simulink model "microgrid"  (R2023b)
settings: Solver=VariableStepAuto  StartTime=0.0  StopTime=24*60*60  RelTol=1e-3
PreLoadFcn:
  | microgrid_parameters
values from neighbouring files (symbols this model uses):
  PV = photovoltaic_parameters    [microgrid_parameters.m]
undefined symbols (not defined in the file or in its folder): BUS, URFC
libraries: fl_lib x19, ee_lib x5, nesl_utility x4, SignalEditorBlockLib x1
settings Model: Creator=michaelfsb  LastModifiedBy=michaelfsb
settings DebuggingCC: IgnoredZcDiagnostic=error

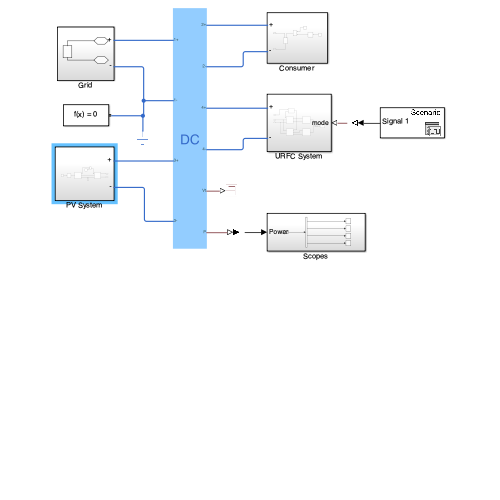
[thumbnail: Simulink's stored preview of the top-level diagram]
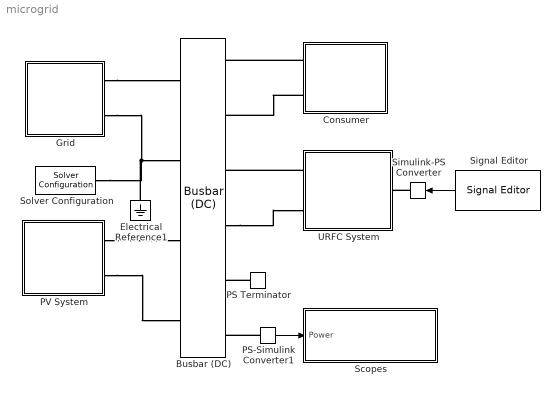
== system microgrid ==
  Busbar (DC) : ee_lib/Connectors & References/Busbar (DC)  n_nodes=ee.enum.connectors.busbar_number_of_connections.four  VRated=BUS.Voltage V  measurement_type=ee.enum.measurementType.instantaneous  averaging_period=1e-2 s  show_ps=ee.enum.connectors.busbar_measurement.true
      settings: InternalSimscapePortConfiguration="{\"Bottom\":[],\"Left\":[{\"id\":\"p1\",\"label\":\"1+\",\"type\":\"foundation.electrical.electrical\"},{\"id\":\"n1\",\"label\":\"1-\",\"type\":\"foundation.electrical.electrical\"},{\"id\":\"p3\",\"label\":\"3+\",\"type\":\"foundation.electrical.electrical\"},{\"id\":\"n3\",\"label\":\"3-\",\"type\":\"foundation.electrical.electrical\"}],\"Right\":[{\"id\":\"p2\",\"label\":\"2+\",\"type\":\"foundation.electrical.electrical\"},{\"id\":\"n2\",\"label\":\"2-\",\"type\":\"foundation.electrical.electrical\"},{\"id\":\"p4\",\"label\":\"4+\",\"type\":\"foundation.electrical.electrical\"},{\"id\":\"n4\",\"label\":\"4-\",\"type\":\"foundation.electrical.electrical\"},{\"id\":\"Vt_ps\",\"label\":\"Vt\",\"type\":\"output\"},{\"id\":\"P4_ps\",\"label\":\"P\",\"type\":\"output\"}],\"Top\":[]}"
  Consumer : Subsystem
  Electrical Reference1 : fl_lib/Electrical/Electrical Elements/Electrical Reference
  Grid : Subsystem
      settings: PortSchema="{\"entries\":[{\"content\":{\"sides\":[{\"content\":{},\"type\":\"ConnectorPlacement.EquallySpacedRectSide\",\"uuid\":\"7d3e1531-3ac3-48d1-8d53-8dc071a39518\"},{\"content\":{\"side\":\"RIGHT\"},\"type\":\"ConnectorPlacement.EquallySpacedRectSide\",\"uuid\":\"25b50bd9-2b9f-4527-8fc7-8205feed0a4d\"},{\"content\":{\"connectorIds\":[\"LConn1\",\"LConn2\"],\"side\":\"TOP\"},\"type\":\"ConnectorPlacement.EquallySpacedRectSide\",\"uuid\":\"ec9d499b-92d3-45f6-91a8-3c7a2a7323b8\"}]},\"type\":\"ConnectorPlacement.EquallySpacedConnector\",\"uuid\":\"21f9d016-eefb-40e7-aeda-3b0d2900fe93\"}],\"packageUris\":[\"http://schema.mathworks.com/mf0/Connector/R2020b\"],\"version\":\"1.0\"}"
  PS Terminator : fl_lib/Physical Signals/Sinks/PS Terminator
  PS-Simulink Converter1 : nesl_utility/PS-Simulink Converter  PhysicalDomain=network_engine_domain  SubClassName=ps_output  LeftPortType=input  RightPortType=output  PseudoPeriodic=off  Frequencies=[]  VectorFormat=inherit  Unit=inherit  AffineConversion=off
  PV System : Subsystem
      settings: PortSchema="{\"entries\":[{\"content\":{\"sides\":[{\"content\":{},\"type\":\"ConnectorPlacement.EquallySpacedRectSide\",\"uuid\":\"7d3e1531-3ac3-48d1-8d53-8dc071a39518\"},{\"content\":{\"side\":\"RIGHT\"},\"type\":\"ConnectorPlacement.EquallySpacedRectSide\",\"uuid\":\"25b50bd9-2b9f-4527-8fc7-8205feed0a4d\"},{\"content\":{\"connectorIds\":[\"LConn1\",\"LConn2\"],\"side\":\"TOP\"},\"type\":\"ConnectorPlacement.EquallySpacedRectSide\",\"uuid\":\"ec9d499b-92d3-45f6-91a8-3c7a2a7323b8\"}]},\"type\":\"ConnectorPlacement.EquallySpacedConnector\",\"uuid\":\"21f9d016-eefb-40e7-aeda-3b0d2900fe93\"}],\"packageUris\":[\"http://schema.mathworks.com/mf0/Connector/R2020b\"],\"version\":\"1.0\"}"
  Scopes : Subsystem
  Signal Editor : SignalEditorBlockLib/Signal Editor  FileName=op_mode_siginal.mat  ActiveScenario=Scenario  ActiveSignal=Signal 1  IsBus=off  OutputBusObjectStr=Bus: BusObject  SampleTime=0  Interpolate=off  ZeroCross=off  OutputAfterFinalValue=Setting to zero  Unit=inherit  PreserveSignalName=on  ApplySigPropsToAllScenarios=on  ApplySigPropsToAllSignals=off
  Simulink-PS Converter : nesl_utility/Simulink-PS Converter  PhysicalDomain=network_engine_domain  SubClassName=ps_input  LeftPortType=input  RightPortType=output  PseudoPeriodic=off  Frequencies=[]  NoiseDistribution=none  NoiseParameters=[]  Unit=1  AffineConversion=off  FilteringAndDerivatives=provide  SimscapeFilterOrder=1  InputFilterTimeConstant=0.001  UdotUserProvided=0
  Solver Configuration : nesl_utility/Solver Configuration  PhysicalDomain=network_engine_domain  SubClassName=solver  LeftPortType=input  RightPortType=generic  Tones=[]  Harmonics=[]  SimulateNoise=off  Profile=off  UseLocalSampling=off  EnableSwitchedLinearOptims=on  FrequencyDomain=off  UseCCode=off  RelTol=0.001  AbsTol=0.001  MinStep=1e-09  ToWorkspace=off  RevertToSquareIcSolve=off  NumHomotopyIterations=100  PhasorMode=off  PhasorModeNumHarmonics=1  ConsistencySolver=NEWTON_XTOL_AFTER_FTOL  IndexReductionMethod=DerivativeReplacement  DoDC=off  ResidualTolerance=1e-09  ConsistencyTolSource=GLOBAL  ConsistencyAbsTol=0.001  ConsistencyRelTol=0.001  ConsistencyTolFactor=0.001  UseLocalSolver=off  LocalSolverChoice=NE_BACKWARD_EULER_ADVANCER  ResolveIndetEquations=on  FunctionEvalNumThread=1  LocalSolverSampleTime=0.001  DoFixedCost=off  MaxNonlinIter=3  MaxModeIter=2  ComputeImpulses=off  ImpulseIterations=2  LinearAlgebra=auto  LinearAlgebraNumThread=0  EquationFormulation=NE_TIME_EF  DelaysMemoryBudget=1024  AutomaticFiltering=on  FilteringTimeConstant=0.001  PartitionStorageMethod=AS_NEEDED  PartitionMemoryBudget=1024  PartitionMethod=ROBUST  MultibodyUseLocalSolver=off  MultibodyLocalSolverChoice=ODE1  MultibodyLocalSolverSampleTime=0.001
  URFC System : Subsystem
  wires:
  PS-Simulink Converter1/1 -> Scopes/1(Power)
  Signal Editor/1 -> Simulink-PS Converter/1
  connections:
  Grid/LConn1 -- Busbar (DC)/LConn1
  PV System/LConn1 -- Busbar (DC)/LConn3
  Consumer/LConn1 -- Busbar (DC)/RConn1
  PV System/LConn2 -- Busbar (DC)/LConn4
  Grid/LConn2 -- Solver Configuration/RConn1 -- Electrical Reference1/LConn1 -- Busbar (DC)/LConn2
  Consumer/LConn2 -- Busbar (DC)/RConn2
  PS-Simulink Converter1/LConn1 -- Busbar (DC)/RConn6
  PS Terminator/LConn1 -- Busbar (DC)/RConn5
  URFC System/RConn1 -- Busbar (DC)/RConn3
  Simulink-PS Converter/RConn1 -- URFC System/LConn1
  Busbar (DC)/RConn4 -- URFC System/RConn2

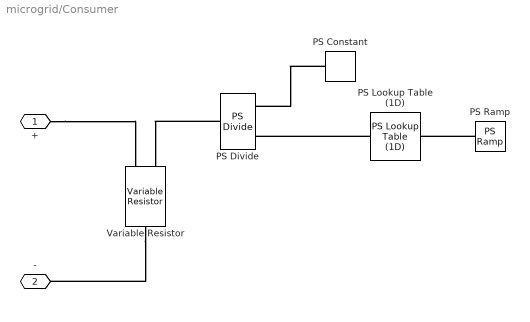
== system microgrid/Consumer ==
  PS Constant : fl_lib/Physical Signals/Sources/PS Constant  constant=BUS.Voltage^2 V^2
  PS Divide : fl_lib/Physical Signals/Functions/PS Divide
  PS Lookup Table (1D) : fl_lib/Physical Signals/Lookup Tables/PS Lookup Table (1D)  x=power_demand.time  f=power_demand.data W  interp_method=simscape.enum.interpolation.linear  extrap_method=simscape.enum.extrapolation.linear
  PS Ramp : fl_lib/Physical Signals/Sources/PS Ramp  slope=1 1/s  start_time=0 s  initial_output=0
  Variable Resistor : fl_lib/Electrical/Electrical Elements/Variable Resistor  Rmin=0 Ohm  thermalEnable=false  thermal_mass=1 J/K  i_specify=off  i_priority=None  i=0 A  i_nominal_specify=off  i_nominal_unit=A  i_nominal_value=1  v_specify=off  v_priority=None  v=0 V  v_nominal_specify=off  v_nominal_unit=V  v_nominal_value=1  T_specify=off  T_priority=None  T=300 K  T_nominal_specify=off  T_nominal_unit=K  T_nominal_value=1
  + : PMIOPort  Side=Left
  - : PMIOPort  Port=2  Side=Left
  connections:
  Variable Resistor/RConn1 -- -/RConn1
  PS Ramp/RConn1 -- PS Lookup Table (1D)/LConn1
  PS Constant/RConn1 -- PS Divide/LConn1
  PS Divide/RConn1 -- Variable Resistor/LConn1
  +/RConn1 -- Variable Resistor/LConn2
  PS Lookup Table (1D)/RConn1 -- PS Divide/LConn2

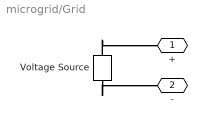
== system microgrid/Grid ==
  Voltage Source : ee_lib/Sources/Voltage Source  dc_voltage=BUS.Voltage V  ac_voltage=0 V  ac_shift=0 rad  ac_frequency=60 Hz  noise_mode=ee.enum.sources.noise.Disabled  PSD=0 V^2/Hz  sample_time=1e-3 s  repeatability=ee.enum.sources.repeatability.NotRepeatable  user_seed=0  auto_seed=414269032  i_specify=off  i_priority=None  i=0 A  i_nominal_specify=off  i_nominal_unit=A  i_nominal_value=1  v_specify=off  v_priority=None  v=0 V  v_nominal_specify=off  v_nominal_unit=V  v_nominal_value=1
  + : PMIOPort  Side=Left
  - : PMIOPort  Port=2  Side=Left
  connections:
  Voltage Source/LConn1 -- +/RConn1
  Voltage Source/RConn1 -- -/RConn1

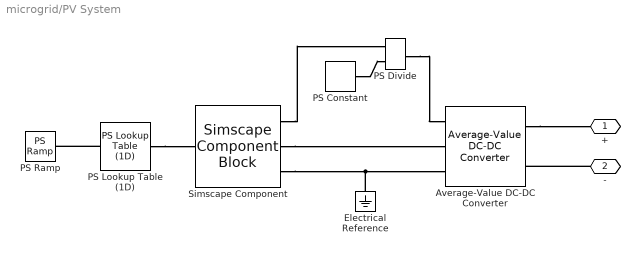
== system microgrid/PV System ==
  Average-Value DC-DC Converter : ee_lib/Semiconductors & Converters/Converters/Average-Value DC-DC Converter  control_option=ee.enum.converters.controlinput.current  converter_type=ee.enum.converters.dcdctype.boost  efficiency_option=ee.enum.converters.efficiency.constant  efficiency_fixed=100  i_vec=[0, 2, 5] A  efficiency_vec=[90, 95, 98]
      settings: InternalSimscapePortConfiguration="{\"Bottom\":[],\"Left\":[{\"id\":\"Iref\",\"label\":\"Iref\",\"type\":\"input\"},{\"id\":\"p1\",\"label\":\"1+\",\"type\":\"foundation.electrical.electrical\"},{\"id\":\"n1\",\"label\":\"1-\",\"type\":\"foundation.electrical.electrical\"}],\"Right\":[{\"id\":\"p2\",\"label\":\"2+\",\"type\":\"foundation.electrical.electrical\"},{\"id\":\"n2\",\"label\":\"2-\",\"type\":\"foundation.electrical.electrical\"}],\"Top\":[]}"
  Electrical Reference : fl_lib/Electrical/Electrical Elements/Electrical Reference
  PS Constant : fl_lib/Physical Signals/Sources/PS Constant  constant=BUS.Voltage V
  PS Divide : fl_lib/Physical Signals/Functions/PS Divide
  PS Lookup Table (1D) : fl_lib/Physical Signals/Lookup Tables/PS Lookup Table (1D)  x=radiation.time  f=radiation.data  interp_method=simscape.enum.interpolation.linear  extrap_method=simscape.enum.extrapolation.linear
  PS Ramp : fl_lib/Physical Signals/Sources/PS Ramp  slope=1 1/s  start_time=0 s  initial_output=0
  Simscape Component : SimscapeComponentBlock  SourceFile=pv_panel  ComponentPath=pv_panel  ComponentVariants="[\"pv_panel\"]"  ComponentVariantNames="[\"pv_panel\"]"  ClassName=pv_panel  SchemaVersion=1  Nps=PV.N_ps  Nss=PV.N_ss  T=PV.T_ps K  Tr=PV.Tr K  Isc=PV.Isc A  Kl=PV.Kl A/K  Ior=PV.Ior A  Ego=PV.Ego V  A=PV.A  v_specify=off  v_priority=None  v=0 V  v_nominal_specify=off  v_nominal_unit=V  v_nominal_value=1  i_specify=off  i_priority=None  i=0 A  i_nominal_specify=off  i_nominal_unit=A  i_nominal_value=1
      settings: CopyFcn=simscape.engine.sli.internal.componentblockcallback(gcbh,'COPY')  PreCopyFcn=simscape.engine.sli.internal.componentblockcallback(gcbh,'PRECOPY')  PreDeleteFcn=simscape.engine.sli.internal.componentblockcallback(gcbh,'PREDELETE')  InternalSimscapePortConfiguration="{\"Bottom\":[],\"Left\":[{\"id\":\"lambda\",\"label\":\"l\",\"type\":\"input\"}],\"Right\":[{\"id\":\"p_mppt\",\"label\":\"p\",\"type\":\"output\"},{\"id\":\"p\",\"label\":\"+\",\"type\":\"foundation.electrical.electrical\"},{\"id\":\"n\",\"label\":\"-\",\"type\":\"foundation.electrical.electrical\"}],\"Top\":[]}"
      mask Type: pv_panel
  + : PMIOPort  Side=Left
  - : PMIOPort  Port=2  Side=Left
  connections:
  Electrical Reference/LConn1 -- Average-Value DC-DC Converter/LConn3 -- Simscape Component/RConn3
  PS Lookup Table (1D)/LConn1 -- PS Ramp/RConn1
  PS Lookup Table (1D)/RConn1 -- Simscape Component/LConn1
  -/RConn1 -- Average-Value DC-DC Converter/RConn2
  Average-Value DC-DC Converter/RConn1 -- +/RConn1
  Simscape Component/RConn2 -- Average-Value DC-DC Converter/LConn2
  Simscape Component/RConn1 -- PS Divide/LConn1
  PS Constant/RConn1 -- PS Divide/LConn2
  PS Divide/RConn1 -- Average-Value DC-DC Converter/LConn1

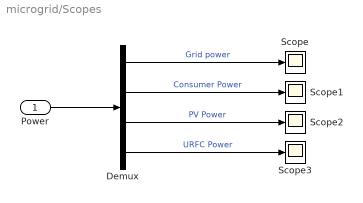
== system microgrid/Scopes ==
  Power : Inport
  Demux : Demux
  Scope{,1..3} (4 alike) : Scope
  wires:
  Power/1 -> Demux/1
  Demux/1 -> Scope/1  "Grid power"
  Demux/4 -> Scope3/1  "URFC Power"
  Demux/2 -> Scope1/1  "Consumer Power"
  Demux/3 -> Scope2/1  "PV Power"

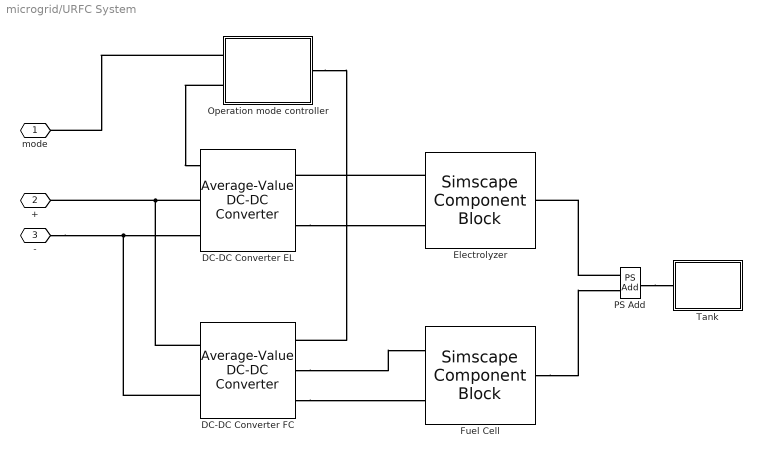
== system microgrid/URFC System ==
  DC-DC Converter EL : ee_lib/Semiconductors & Converters/Converters/Average-Value DC-DC Converter  control_option=ee.enum.converters.controlinput.current  converter_type=ee.enum.converters.dcdctype.buck  efficiency_option=ee.enum.converters.efficiency.constant  efficiency_fixed=100  i_vec=[0, 2, 5] A  efficiency_vec=[90, 95, 98]
      settings: LogSimulationData=on  InternalSimscapePortConfiguration="{\"Bottom\":[],\"Left\":[{\"id\":\"Iref\",\"label\":\"Iref\",\"type\":\"input\"},{\"id\":\"p1\",\"label\":\"1+\",\"type\":\"foundation.electrical.electrical\"},{\"id\":\"n1\",\"label\":\"1-\",\"type\":\"foundation.electrical.electrical\"}],\"Right\":[{\"id\":\"p2\",\"label\":\"2+\",\"type\":\"foundation.electrical.electrical\"},{\"id\":\"n2\",\"label\":\"2-\",\"type\":\"foundation.electrical.electrical\"}],\"Top\":[]}"
  DC-DC Converter FC : ee_lib/Semiconductors & Converters/Converters/Average-Value DC-DC Converter  control_option=ee.enum.converters.controlinput.current  converter_type=ee.enum.converters.dcdctype.buck  efficiency_option=ee.enum.converters.efficiency.constant  efficiency_fixed=100  i_vec=[0, 2, 5] A  efficiency_vec=[90, 95, 98]
      settings: LogSimulationData=on  InternalSimscapePortConfiguration="{\"Bottom\":[],\"Left\":[{\"id\":\"Iref\",\"label\":\"Iref\",\"type\":\"input\"},{\"id\":\"p1\",\"label\":\"1+\",\"type\":\"foundation.electrical.electrical\"},{\"id\":\"n1\",\"label\":\"1-\",\"type\":\"foundation.electrical.electrical\"}],\"Right\":[{\"id\":\"p2\",\"label\":\"2+\",\"type\":\"foundation.electrical.electrical\"},{\"id\":\"n2\",\"label\":\"2-\",\"type\":\"foundation.electrical.electrical\"}],\"Top\":[]}"
  Electrolyzer : SimscapeComponentBlock  SourceFile=urfc_electrolyzer  ComponentPath=urfc_electrolyzer  ComponentVariants="[\"urfc_electrolyzer\"]"  ComponentVariantNames="[\"urfc_electrolyzer\"]"  ClassName=urfc_electrolyzer  SchemaVersion=1  N_cells=10  A_cell=100 cm^2  alpha=0.5  E_rev_0=1.23 V  I_loss_internal=0.008 A/cm^2  I_o_anode=0.15 A/cm^2  I_o_cathode=1.5e-4 A/cm^2  R_ion=0.01 Ohm*cm^2  R_CR=0.03 Ohm*cm^2  R_elect=0 Ohm*cm^2  I_limit_anode=15 A/cm^2  I_limit_cathode=2.5 A/cm^2  A_anodo=0.0304 V  A_catodo=0.0507 V  T=353.15 K  R_gas=8.3145 J/(K*mol)  F_constant=96485 C/mol  n_electrons=2  i_specify=off  i_priority=None  i=0 A  i_nominal_specify=off  i_nominal_unit=A  i_nominal_value=1  v_specify=off  v_priority=None  v=0 V  v_nominal_specify=off  v_nominal_unit=V  v_nominal_value=1
      settings: CopyFcn=simscape.engine.sli.internal.componentblockcallback(gcbh,'COPY')  PreCopyFcn=simscape.engine.sli.internal.componentblockcallback(gcbh,'PRECOPY')  PreDeleteFcn=simscape.engine.sli.internal.componentblockcallback(gcbh,'PREDELETE')  InternalSimscapePortConfiguration="{\"Bottom\":[],\"Left\":[{\"id\":\"p\",\"label\":\"+\",\"type\":\"foundation.electrical.electrical\"},{\"id\":\"n\",\"label\":\"-\",\"type\":\"foundation.electrical.electrical\"}],\"Right\":[{\"id\":\"h2\",\"label\":\"H2\",\"type\":\"output\"}],\"Top\":[]}"
      mask Type: Electrolyzer mode model of a URFC
  Fuel Cell : SimscapeComponentBlock  SourceFile=urfc_fuel_cell  ComponentPath=urfc_fuel_cell  ComponentVariants="[\"urfc_fuel_cell\"]"  ComponentVariantNames="[\"urfc_fuel_cell\"]"  ClassName=urfc_fuel_cell  SchemaVersion=1  N_cells=10  A_cell=100 cm^2  alpha=0.5  E_rev_0=1.23 V  I_loss_internal=0.008 A/cm^2  I_o_anode=0.15 A/cm^2  I_o_cathode=1.5e-4 A/cm^2  R_ion=0.01 Ohm*cm^2  R_CR=0.03 Ohm*cm^2  R_elect=0 Ohm*cm^2  I_limit_anode=15 A/cm^2  I_limit_cathode=2.5 A/cm^2  A_anodo=0.0304 V  A_catodo=0.0507 V  T=353.15 K  R_gas=8.3145 J/(K*mol)  F_constant=96485 C/mol  n_electrons=2  i_specify=off  i_priority=None  i=0 A  i_nominal_specify=off  i_nominal_unit=A  i_nominal_value=1  v_specify=off  v_priority=None  v=0 V  v_nominal_specify=off  v_nominal_unit=V  v_nominal_value=1
      settings: CopyFcn=simscape.engine.sli.internal.componentblockcallback(gcbh,'COPY')  PreCopyFcn=simscape.engine.sli.internal.componentblockcallback(gcbh,'PRECOPY')  PreDeleteFcn=simscape.engine.sli.internal.componentblockcallback(gcbh,'PREDELETE')  InternalSimscapePortConfiguration="{\"Bottom\":[],\"Left\":[{\"id\":\"p\",\"label\":\"+\",\"type\":\"foundation.electrical.electrical\"},{\"id\":\"n\",\"label\":\"-\",\"type\":\"foundation.electrical.electrical\"}],\"Right\":[{\"id\":\"h2\",\"label\":\"H2\",\"type\":\"output\"}],\"Top\":[]}"
      mask Type: Fuel Cell mode model of a URFC
  Operation mode controller : Subsystem
  PS Add : fl_lib/Physical Signals/Functions/PS Add
  Tank : Subsystem
  mode : PMIOPort  Side=Left
  + : PMIOPort  Port=2  Side=Right
  - : PMIOPort  Port=3  Side=Right
  connections:
  DC-DC Converter EL/RConn2 -- Electrolyzer/LConn2
  -/RConn1 -- DC-DC Converter FC/RConn2 -- DC-DC Converter EL/LConn3
  Electrolyzer/LConn1 -- DC-DC Converter EL/RConn1
  DC-DC Converter EL/LConn2 -- DC-DC Converter FC/RConn1 -- +/RConn1
  PS Add/RConn1 -- Tank/LConn1
  PS Add/LConn1 -- Electrolyzer/RConn1
  Fuel Cell/RConn1 -- PS Add/LConn2
  DC-DC Converter FC/LConn2 -- Fuel Cell/LConn1
  DC-DC Converter FC/LConn3 -- Fuel Cell/LConn2
  Operation mode controller/LConn1 -- mode/RConn1
  Operation mode controller/LConn2 -- DC-DC Converter EL/LConn1
  Operation mode controller/RConn1 -- DC-DC Converter FC/LConn1

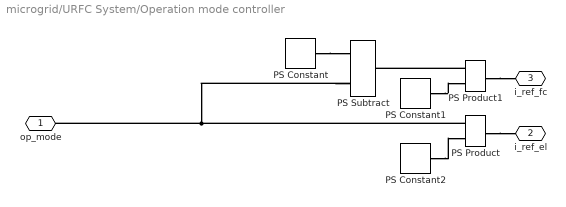
== system microgrid/URFC System/Operation mode controller ==
  PS Constant : fl_lib/Physical Signals/Sources/PS Constant  constant=1
  PS Constant1 : fl_lib/Physical Signals/Sources/PS Constant  constant=URFC.FuelCell.i_op/3 A
  PS Constant2 : fl_lib/Physical Signals/Sources/PS Constant  constant=URFC.Electrolyzer.i_op A
  PS Product : fl_lib/Physical Signals/Functions/PS Product
  PS Product1 : fl_lib/Physical Signals/Functions/PS Product
  PS Subtract : fl_lib/Physical Signals/Functions/PS Subtract
  op_mode : PMIOPort  Side=Left
  i_ref_el : PMIOPort  Port=2  Side=Left
  i_ref_fc : PMIOPort  Port=3  Side=Right
  connections:
  PS Product/RConn1 -- i_ref_el/RConn1
  PS Constant/RConn1 -- PS Subtract/LConn1
  PS Product1/RConn1 -- i_ref_fc/RConn1
  PS Product/LConn1 -- op_mode/RConn1 -- PS Subtract/LConn2
  PS Product1/LConn1 -- PS Subtract/RConn1
  PS Constant1/RConn1 -- PS Product1/LConn2
  PS Constant2/RConn1 -- PS Product/LConn2

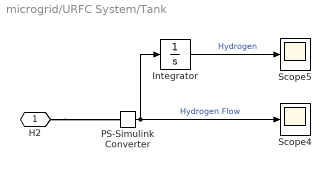
== system microgrid/URFC System/Tank ==
  Integrator : Integrator  InitialCondition=URFC.Tank.Initial
  PS-Simulink Converter : nesl_utility/PS-Simulink Converter  PhysicalDomain=network_engine_domain  SubClassName=ps_output  LeftPortType=input  RightPortType=output  PseudoPeriodic=off  Frequencies=[]  VectorFormat=inherit  Unit=inherit  AffineConversion=off
  Scope4 : Scope
  Scope5 : Scope
  H2 : PMIOPort  Side=Left
  wires:
  Integrator/1 -> Scope5/1  "Hydrogen"
  PS-Simulink Converter/1 -> Integrator/1, Scope4/1  "Hydrogen Flow"
  connections:
  H2/RConn1 -- PS-Simulink Converter/LConn1
